simulink model "SensorCalibration"  (R2018b)
settings: configuration reference "RPi_ControlRate" (kept outside this file)
values from neighbouring files (symbols this model uses):
  AccelIIR_Den = [1.000000000000000  -1.561018075800718   0.641351538057563]    [loadSensorData.m]
  AccelIIR_Num = [0.020083365564211   0.040166731128423   0.020083365564211]    [loadSensorData.m]
  controlRate = 0.025    [loadBusData.m]
  M_IMU_To_Body = ZRot(pi)*EulerToDCM_321(Euler_IMU_To_Body)    [loadSensorData.m]
  NorthAngle = -84*dtr    (= -1.46607657168)    [loadSensorData.m]
undefined symbols (not defined in the file or in its folder): DiscIntNeverNeededParam
settings Model: EnablePacing=on  Creator=barthal  LastModifiedBy=barthal
settings ConfigSetRef: SourceLocation=Base Workspace

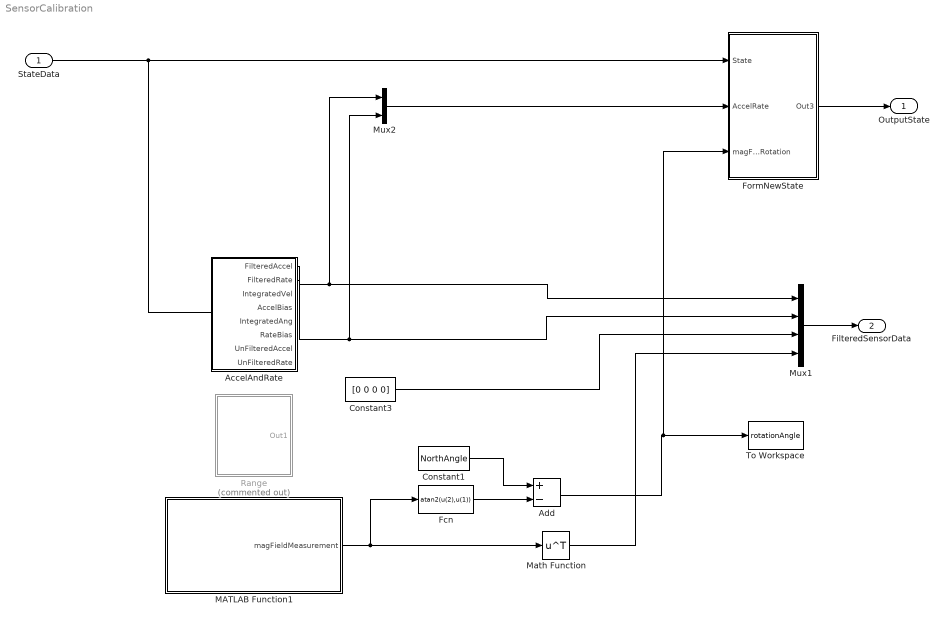
== system SensorCalibration ==
  StateData : Inport  OutDataTypeStr=Bus: FullStateBus
  AccelAndRate : Subsystem
  Add : Sum  Inputs=+-
  Constant1 : Constant  Value=NorthAngle
  Constant3 : Constant  Value=[0 0 0 0]
  Fcn : Fcn  Expr=atan2(u(2),u(1))
  FormNewState : Subsystem
  MATLAB Function1 : MATLAB Function  TreatAsAtomicUnit=on
  Math Function : Math  Operator=transpose  SaturateOnIntegerOverflow=on
  Mux1 : Mux
  Mux2 : Mux  Inputs=2
  Range : Subsystem  Commented=on
  To Workspace : ToWorkspace  VariableName=rotationAngle  SaveFormat=Timeseries  SampleTime=-1
  OutputState : Outport  OutDataTypeStr=Bus: FullStateBus
  FilteredSensorData : Outport  Port=2
  wires:
  AccelAndRate/2(FilteredRate) -> Mux2/2, Mux1/2
  AccelAndRate/1(FilteredAccel) -> Mux2/1, Mux1/1
  Mux1/1 -> FilteredSensorData/1
  Constant3/1 -> Mux1/3
  MATLAB Function1/1(magFieldMeasurement) -> Fcn/1, Math Function/1
  Math Function/1 -> Mux1/4
  Add/1 -> FormNewState/3(magFieldRotation), To Workspace/1
  Constant1/1 -> Add/1
  Fcn/1 -> Add/2
  StateData/1 -> FormNewState/1(State)
  Mux2/1 -> FormNewState/2(AccelRate)
  FormNewState/1(Out3) -> OutputState/1

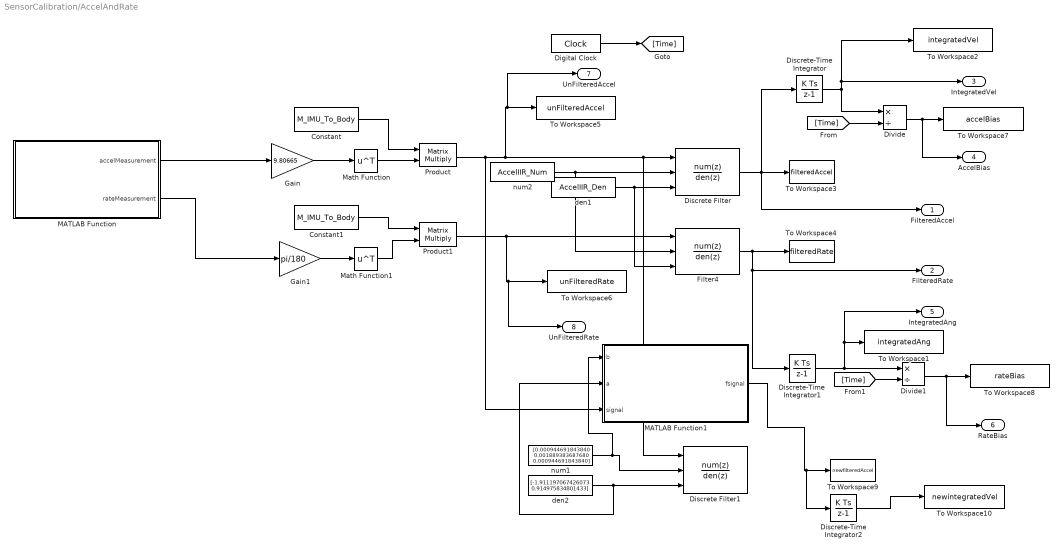
== system SensorCalibration/AccelAndRate ==
  Constant : Constant  Value=M_IMU_To_Body
  Constant1 : Constant  Value=M_IMU_To_Body
  Digital Clock : DigitalClock  SampleTime=controlRate
  Discrete Filter : DiscreteFilter  NumeratorSource=Input port  DenominatorSource=Input port  a0EqualsOne=on
      settings: InputPortMap=u0,p1,p3
  Discrete Filter1 : DiscreteFilter  NumeratorSource=Input port  DenominatorSource=Input port  a0EqualsOne=on
      settings: InputPortMap=u0,p1,p3
  Discrete-Time Integrator : DiscreteIntegrator  SampleTime=-1  ICPrevOutput=DiscIntNeverNeededParam  ICPrevScaledInput=DiscIntNeverNeededParam
  Discrete-Time Integrator1 : DiscreteIntegrator  SampleTime=-1  ICPrevOutput=DiscIntNeverNeededParam  ICPrevScaledInput=DiscIntNeverNeededParam
  Discrete-Time Integrator2 : DiscreteIntegrator  SampleTime=-1  ICPrevOutput=DiscIntNeverNeededParam  ICPrevScaledInput=DiscIntNeverNeededParam
  Divide : Product  Inputs=*/
  Divide1 : Product  Inputs=*/
  Filter4 : DiscreteFilter  Tag=BlockMethodSubSystem  NumeratorSource=Input port  Numerator=[2.46193004641406277e-06 4.92386009282812554e-06 2.46193004641406277e-06]  DenominatorSource=Input port  Denominator=[1 -1.99555712434578902 0.995566972065974776]  a0EqualsOne=on
      settings: InputPortMap=u0,p1,p3
  Gain : Gain  Gain=9.80665
  Gain1 : Gain  Gain=pi/180
  MATLAB Function : MATLAB Function  TreatAsAtomicUnit=on
  MATLAB Function1 : MATLAB Function  TreatAsAtomicUnit=on
  Math Function : Math  Operator=transpose  SaturateOnIntegerOverflow=on
  Math Function1 : Math  Operator=transpose  SaturateOnIntegerOverflow=on
  Product : Product  Multiplication=Matrix(*)
  Product1 : Product  Multiplication=Matrix(*)
  To Workspace1 : ToWorkspace  VariableName=integratedAng  SaveFormat=Timeseries  SampleTime=-1
  To Workspace10 : ToWorkspace  VariableName=newintegratedVel  SaveFormat=Timeseries  SampleTime=-1
  To Workspace2 : ToWorkspace  VariableName=integratedVel  SaveFormat=Timeseries  SampleTime=-1
  To Workspace3 : ToWorkspace  VariableName=filteredAccel  SaveFormat=Timeseries  SampleTime=-1
  To Workspace4 : ToWorkspace  VariableName=filteredRate  SaveFormat=Timeseries  SampleTime=-1
  To Workspace5 : ToWorkspace  VariableName=unFilteredAccel  SaveFormat=Timeseries  SampleTime=-1
  To Workspace6 : ToWorkspace  VariableName=unFilteredRate  SaveFormat=Timeseries  SampleTime=-1
  To Workspace7 : ToWorkspace  VariableName=accelBias  SaveFormat=Timeseries  SampleTime=-1
  To Workspace8 : ToWorkspace  VariableName=rateBias  SaveFormat=Timeseries  SampleTime=-1
  To Workspace9 : ToWorkspace  VariableName=newfilteredAccel  SaveFormat=Timeseries  SampleTime=-1
  den1 : Constant  Value=AccelIIR_Den
  den2 : Constant  Value="[-1.911197067426073   0.914975834801433]"
  num1 : Constant  Value="[0.000944691843840   0.001889383687680   0.000944691843840]"  VectorParams1D=off
  num2 : Constant  Value=AccelIIR_Num  VectorParams1D=off
  FilteredAccel : Outport
  FilteredRate : Outport  Port=2
  IntegratedVel : Outport  Port=3
  AccelBias : Outport  Port=4
  IntegratedAng : Outport  Port=5
  RateBias : Outport  Port=6
  UnFilteredAccel : Outport  Port=7
  UnFilteredRate : Outport  Port=8
  wires:
  Product/1 -> Discrete Filter1/1, Discrete Filter/1, UnFilteredAccel/1, To Workspace5/1, MATLAB Function1/3(signal)
  Discrete Filter/1 -> Discrete-Time Integrator/1, FilteredAccel/1, To Workspace3/1
  Product1/1 -> UnFilteredRate/1, To Workspace6/1, Filter4/1
  Filter4/1 -> Discrete-Time Integrator1/1, FilteredRate/1, To Workspace4/1
  MATLAB Function/2(rateMeasurement) -> Gain1/1
  MATLAB Function/1(accelMeasurement) -> Gain/1
  Gain/1 -> Math Function/1
  Constant/1 -> Product/1
  Constant1/1 -> Product1/1
  Gain1/1 -> Math Function1/1
  Math Function/1 -> Product/2
  Math Function1/1 -> Product1/2
  den1/1 -> Filter4/3, Discrete Filter/3
  Discrete-Time Integrator/1 -> IntegratedVel/1, To Workspace2/1, Divide/1
  Divide/1 -> AccelBias/1, To Workspace7/1
  Discrete-Time Integrator1/1 -> IntegratedAng/1, To Workspace1/1, Divide1/1
  Digital Clock/1 -> [Time]
  [Time] -> Divide/2
  [Time] -> Divide1/2
  Divide1/1 -> RateBias/1, To Workspace8/1
  num1/1 -> MATLAB Function1/1(b), Discrete Filter1/2
  den2/1 -> MATLAB Function1/2(a), Discrete Filter1/3
  Discrete-Time Integrator2/1 -> To Workspace10/1
  num2/1 -> Filter4/2, Discrete Filter/2
  MATLAB Function1/1(fsignal) -> Discrete-Time Integrator2/1, To Workspace9/1

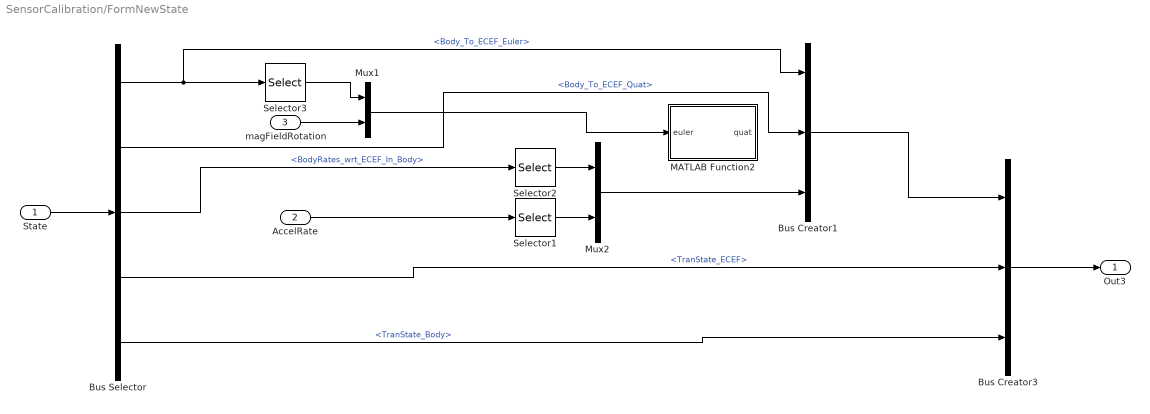
== system SensorCalibration/FormNewState ==
  State : Inport
  AccelRate : Inport  Port=2
  magFieldRotation : Inport  Port=3
  Bus Creator1 : BusCreator  Inputs=3  OutDataTypeStr=Bus: RotStateBodyECEFBus
      settings: InheritFromInputs=off
  Bus Creator3 : BusCreator  Inputs=3  OutDataTypeStr=Bus: FullStateBus
      settings: InheritFromInputs=off
  Bus Selector : BusSelector  OutputSignals=RotState_Body_ECEF.Body_To_ECEF_Euler,RotState_Body_ECEF.Body_To_ECEF_Quat,RotState_Body_ECEF.BodyRates_wrt_ECEF_In_Body,TranState_ECEF,TranState_Body
  MATLAB Function2 : MATLAB Function  TreatAsAtomicUnit=on
  Mux1 : Mux  Inputs=2
  Mux2 : Mux  Inputs=2
  Selector1 : Selector  InputPortWidth=6  IndexOptions=Index vector (dialog)  Indices=[6]  OutputSizes=1
  Selector2 : Selector  InputPortWidth=3  IndexOptions=Index vector (dialog)  Indices=[1:2]  OutputSizes=1
  Selector3 : Selector  InputPortWidth=3  IndexOptions=Index vector (dialog)  Indices=[1:2]  OutputSizes=1
  Out3 : Outport
  wires:
  State/1 -> Bus Selector/1
  Selector2/1 -> Mux2/1
  Bus Selector/3 -> Selector2/1  "<BodyRates_wrt_ECEF_In_Body>"
  Selector1/1 -> Mux2/2
  Bus Selector/5 -> Bus Creator3/3  "<TranState_Body>"
  AccelRate/1 -> Selector1/1
  Bus Selector/4 -> Bus Creator3/2  "<TranState_ECEF>"
  Bus Creator3/1 -> Out3/1
  Mux2/1 -> Bus Creator1/3
  Bus Selector/1 -> Bus Creator1/1, Selector3/1  "<Body_To_ECEF_Euler>"
  Selector3/1 -> Mux1/1
  magFieldRotation/1 -> Mux1/2
  Mux1/1 -> MATLAB Function2/1(euler)
  Bus Creator1/1 -> Bus Creator3/1
  Bus Selector/2 -> Bus Creator1/2  "<Body_To_ECEF_Quat>"

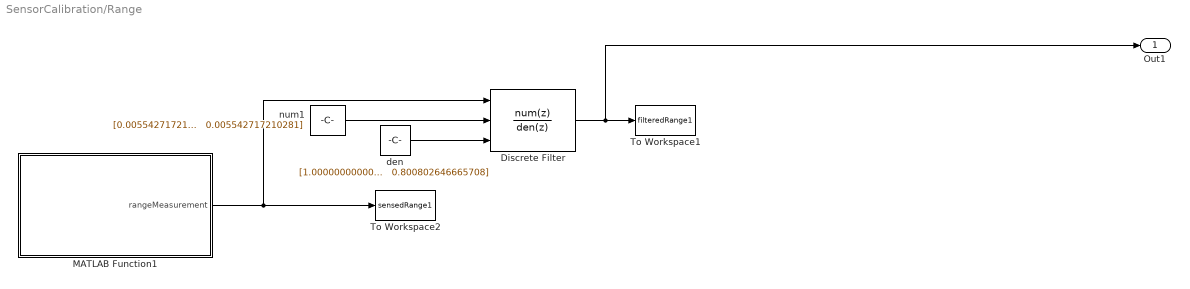
== system SensorCalibration/Range ==
  Discrete Filter : DiscreteFilter  NumeratorSource=Input port  DenominatorSource=Input port  a0EqualsOne=on
      settings: InputPortMap=u0,p1,p3
  MATLAB Function1 : MATLAB Function  TreatAsAtomicUnit=on
  To Workspace1 : ToWorkspace  VariableName=filteredRange1  SaveFormat=Timeseries  SampleTime=-1
  To Workspace2 : ToWorkspace  VariableName=sensedRange1  SaveFormat=Timeseries  SampleTime=-1
  den : Constant  Value="[1.000000000000000  -1.778631777824585   0.800802646665708]"
  num1 : Constant  Value="[0.005542717210281   0.011085434420561   0.005542717210281]"  VectorParams1D=off
  Out1 : Outport
  wires:
  MATLAB Function1/1(rangeMeasurement) -> To Workspace2/1, Discrete Filter/1
  Discrete Filter/1 -> Out1/1, To Workspace1/1
  den/1 -> Discrete Filter/3
  num1/1 -> Discrete Filter/2

== matlab function SensorCalibration/MATLAB Function1 ==
  data: magFieldMeasurement output
function magFieldMeasurement  = callgetMagPhidgetData()

% These variables must be persistent to ensure the attachment to the
% sensor channel is maintained
persistent magPhidget

% Not all python functions seem to be able to be called from a Matlab 
% function block, so the entire function is considered extrinsic
coder.extrinsic('getMagnetometerPhidgetData');
coder.extrinsic('py.Magnetometer.Magnetometer');

% Create the channel to the sensor
% This code needs error handling
if isempty(magPhidget)
    magPhidget = py.Magnetometer.Magnetometer;
end

% The data types need to be pre-allocated
magFieldMeasurement = [0 0 0];
magTimestamp = 0;

% Get the sensor data
[magFieldMeasurement,magTimestamp] = getMagnetometerPhidgetData(magPhidget);

== matlab function SensorCalibration/AccelAndRate/MATLAB Function1 ==
  data: fsignal output; b input; a input; signal input
function fsignal = callfiltfilt(b,a,signal)

fsignal = filtfilt(b,a,signal);

== matlab function SensorCalibration/FormNewState/MATLAB Function2 ==
  data: quat output; euler input
function quat  = computeQuat(euler)

quat = euler2quat(euler);

== matlab function SensorCalibration/AccelAndRate/MATLAB Function ==
  data: accelMeasurement output; rateMeasurement output
function [accelMeasurement,rateMeasurement]= callgetAccelPhidgetData()

% These variables must be persistent to ensure the attachment to the
% sensor channel is maintained
persistent accelPhidget gyroPhidget 

% Not all python functions seem to be able to be called from a Matlab 
% function block, so the entire function is considered extrinsic
coder.extrinsic('getAccelPhidgetData');
coder.extrinsic('py.Accelerometer.Accelerometer');
coder.extrinsic('py.Gyroscope.Gyroscope');

% Create the channel to the sensor
% This code needs error handling
if isempty(accelPhidget)
    accelPhidget = py.Accelerometer.Accelerometer;
end
if isempty(gyroPhidget)
    gyroPhidget = py.Gyroscope.Gyroscope;
end

% The data types need to be pre-allocated
accelMeasurement = [0 0 0];
rateMeasurement = [0 0 0];
accelTimestamp = 0;
rateTimestamp = 0;

% Get the sensor data
[accelMeasurement,rateMeasurement,accelTimestamp,rateTimestamp] = getAccelPhidgetData(accelPhidget,gyroPhidget);

== matlab function SensorCalibration/Range/MATLAB Function1 ==
  data: rangeMeasurement output
function rangeMeasurement  = callgetRangePhidgetData()

% These variables must be persistent to ensure the attachment to the
% sensor channel is maintained
persistent rangePhidget1 rangePhidget2 rangePhidget3 rangePhidget4

% Not all python functions seem to be able to be called from a Matlab 
% function block, so the entire function is considered extrinsic
coder.extrinsic('getRangePhidgetData');
coder.extrinsic('py.DistanceSensor.DistanceSensor');

% Create the channel to the sensor
% This code needs error handling
if isempty(rangePhidget1)
    rangePhidget1 = py.DistanceSensor.DistanceSensor;
end
if isempty(rangePhidget2)
    rangePhidget2 = py.DistanceSensor.DistanceSensor;
end
if isempty(rangePhidget3)
    rangePhidget3 = py.DistanceSensor.DistanceSensor;
end
if isempty(rangePhidget4)
    rangePhidget4 = py.DistanceSensor.DistanceSensor;
end

% The data types need to be pre-allocated
rangeMeasurement = [0 0 0 0];

% Get the sensor data
[rangeMeasurement] = getRangePhidgetData(rangePhidget1,rangePhidget2,rangePhidget3,rangePhidget4);
